simulink model "code_gen_man_bin"  (Simulink 7.5)
settings: Solver=FixedStepDiscrete  SolverMode=SingleTasking  StartTime=0.0  StopTime=10.0  FixedStep=0.01  RelTol=1e-3
InitFcn:
  | boat_constants
values from neighbouring files (symbols this model uses):
  figure8_waypoints = int32([ ... (first row only)    [boat_constants.m]
  InitialPoint = 0    [boat_constants.m]    (also in l2plus.m)
  IPStar = 0    [boat_constants.m]    (also in l2plus.m)
  ISA_g = 9.815    [boat_constants.m]
  MaxDwnPthStar = 1    [boat_constants.m]    (also in l2plus.m)
  OC2max = 49999    [boat_constants.m]    (also in simulation_constants.m)
  sampling_waypoints = int32([ ... (first row only)    [boat_constants.m]
  switchDistance = 4    [boat_constants.m]    (also in l2plus.m)
  T_step = 0.01    [boat_constants.m]    (also in common.m)
  tanIntercept = tan( 45*pi/180 )    [boat_constants.m]    (also in l2plus.m)
  test_waypoints = int32([ ... (first row only)    [boat_constants.m]
  TStar = single(4.5)    [boat_constants.m]    (also in l2plus.m = single(2))
  Turn2Track = 0    [boat_constants.m]    (also in l2plus.m)
  wheelbase = 3.27    [boat_constants.m]
undefined symbols (not defined in the file or in its folder): clearGpsData, clearSensorData, cpInitCommunications, DataEEInitAndClear, DataEEWrite, DiscIntNeverNeededParam, ecan1_buffered_transmit_matlab, ecan1_error_status_matlab, ecan1_init, GetAirData, getGpsData, getRevoData, getSensorData, GetThrottleData, GetWaterData, GetWindData, Init_onlyOnce, Init_Reset, initCalibrationRange, initGps, processNewCommData, processNewGpsData, processNewRevoData, setHilMode, u1, u2, uart1EnqueueStateData, uart2EnqueueActuatorData, y1
libraries: simulink x80, dsPICdrivers x50, uSimLib x4, simulink_need_slupdate x4
(part 2 of 6)

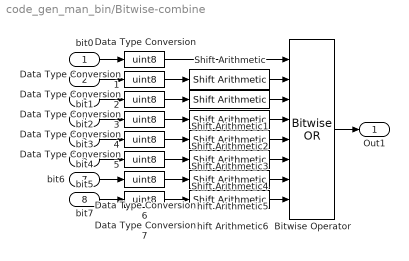
== system code_gen_man_bin/Bitwise-combine ==
  bit0 : Inport
  bit1 : Inport  Port=2
  bit2 : Inport  Port=3
  bit3 : Inport  Port=4
  bit4 : Inport  Port=5
  bit5 : Inport  Port=6
  bit6 : Inport  Port=7
  bit7 : Inport  Port=8
  Bitwise Operator : simulink/Logic and Bit Operations/Bitwise Operator  logicop=OR  UseBitMask=off  NumInputPorts=8  BitMask=bin2dec('11011001')  BitMaskRealWorld=Stored Integer
  Data Type Conversion{,1..7} (8 alike) : DataTypeConversion  OutDataTypeMode=uint8  OutDataType=fixdt(1, 16)  OutScaling=2^0  OutDataTypeStr=uint8
  Shift Arithmetic : simulink/Logic and Bit Operations/Shift Arithmetic  SystemSampleTime=-1  nBitShiftRight=-1  nBinPtShiftRight=0
  Shift Arithmetic1 : simulink/Logic and Bit Operations/Shift Arithmetic  SystemSampleTime=-1  nBitShiftRight=-2  nBinPtShiftRight=0
  Shift Arithmetic2 : simulink/Logic and Bit Operations/Shift Arithmetic  SystemSampleTime=-1  nBitShiftRight=-3  nBinPtShiftRight=0
  Shift Arithmetic3 : simulink/Logic and Bit Operations/Shift Arithmetic  SystemSampleTime=-1  nBitShiftRight=-4  nBinPtShiftRight=0
  Shift Arithmetic4 : simulink/Logic and Bit Operations/Shift Arithmetic  SystemSampleTime=-1  nBitShiftRight=-5  nBinPtShiftRight=0
  Shift Arithmetic5 : simulink/Logic and Bit Operations/Shift Arithmetic  SystemSampleTime=-1  nBitShiftRight=-6  nBinPtShiftRight=0
  Shift Arithmetic6 : simulink/Logic and Bit Operations/Shift Arithmetic  SystemSampleTime=-1  nBitShiftRight=-7  nBinPtShiftRight=0
  Out1 : Outport
  wires:
  Shift Arithmetic/1 -> Bitwise Operator/2
  Shift Arithmetic1/1 -> Bitwise Operator/3
  Shift Arithmetic2/1 -> Bitwise Operator/4
  Data Type Conversion/1 -> Bitwise Operator/1
  Data Type Conversion1/1 -> Shift Arithmetic/1
  Data Type Conversion2/1 -> Shift Arithmetic1/1
  Data Type Conversion3/1 -> Shift Arithmetic2/1
  Data Type Conversion4/1 -> Shift Arithmetic3/1
  Shift Arithmetic3/1 -> Bitwise Operator/5
  Data Type Conversion5/1 -> Shift Arithmetic4/1
  Data Type Conversion6/1 -> Shift Arithmetic5/1
  Shift Arithmetic4/1 -> Bitwise Operator/6
  Shift Arithmetic5/1 -> Bitwise Operator/7
  Data Type Conversion7/1 -> Shift Arithmetic6/1
  Shift Arithmetic6/1 -> Bitwise Operator/8
  bit0/1 -> Data Type Conversion/1
  bit1/1 -> Data Type Conversion1/1
  bit2/1 -> Data Type Conversion2/1
  bit3/1 -> Data Type Conversion3/1
  Bitwise Operator/1 -> Out1/1
  bit4/1 -> Data Type Conversion4/1
  bit5/1 -> Data Type Conversion5/1
  bit6/1 -> Data Type Conversion6/1
  bit7/1 -> Data Type Conversion7/1

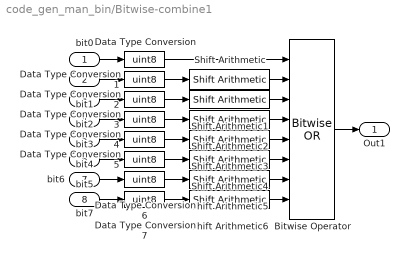
== system code_gen_man_bin/Bitwise-combine1 ==
  bit0 : Inport
  bit1 : Inport  Port=2
  bit2 : Inport  Port=3
  bit3 : Inport  Port=4
  bit4 : Inport  Port=5
  bit5 : Inport  Port=6
  bit6 : Inport  Port=7
  bit7 : Inport  Port=8
  Bitwise Operator : simulink/Logic and Bit Operations/Bitwise Operator  logicop=OR  UseBitMask=off  NumInputPorts=8  BitMask=bin2dec('11011001')  BitMaskRealWorld=Stored Integer
  Data Type Conversion{,1..7} (8 alike) : DataTypeConversion  OutDataTypeMode=uint8  OutDataType=fixdt(1, 16)  OutScaling=2^0  OutDataTypeStr=uint8
  Shift Arithmetic : simulink/Logic and Bit Operations/Shift Arithmetic  SystemSampleTime=-1  nBitShiftRight=-1  nBinPtShiftRight=0
  Shift Arithmetic1 : simulink/Logic and Bit Operations/Shift Arithmetic  SystemSampleTime=-1  nBitShiftRight=-2  nBinPtShiftRight=0
  Shift Arithmetic2 : simulink/Logic and Bit Operations/Shift Arithmetic  SystemSampleTime=-1  nBitShiftRight=-3  nBinPtShiftRight=0
  Shift Arithmetic3 : simulink/Logic and Bit Operations/Shift Arithmetic  SystemSampleTime=-1  nBitShiftRight=-4  nBinPtShiftRight=0
  Shift Arithmetic4 : simulink/Logic and Bit Operations/Shift Arithmetic  SystemSampleTime=-1  nBitShiftRight=-5  nBinPtShiftRight=0
  Shift Arithmetic5 : simulink/Logic and Bit Operations/Shift Arithmetic  SystemSampleTime=-1  nBitShiftRight=-6  nBinPtShiftRight=0
  Shift Arithmetic6 : simulink/Logic and Bit Operations/Shift Arithmetic  SystemSampleTime=-1  nBitShiftRight=-7  nBinPtShiftRight=0
  Out1 : Outport
  wires:
  Shift Arithmetic/1 -> Bitwise Operator/2
  Shift Arithmetic1/1 -> Bitwise Operator/3
  Shift Arithmetic2/1 -> Bitwise Operator/4
  Data Type Conversion/1 -> Bitwise Operator/1
  Data Type Conversion1/1 -> Shift Arithmetic/1
  Data Type Conversion2/1 -> Shift Arithmetic1/1
  Data Type Conversion3/1 -> Shift Arithmetic2/1
  Data Type Conversion4/1 -> Shift Arithmetic3/1
  Shift Arithmetic3/1 -> Bitwise Operator/5
  Data Type Conversion5/1 -> Shift Arithmetic4/1
  Data Type Conversion6/1 -> Shift Arithmetic5/1
  Shift Arithmetic4/1 -> Bitwise Operator/6
  Shift Arithmetic5/1 -> Bitwise Operator/7
  Data Type Conversion7/1 -> Shift Arithmetic6/1
  Shift Arithmetic6/1 -> Bitwise Operator/8
  bit0/1 -> Data Type Conversion/1
  bit1/1 -> Data Type Conversion1/1
  bit2/1 -> Data Type Conversion2/1
  bit3/1 -> Data Type Conversion3/1
  Bitwise Operator/1 -> Out1/1
  bit4/1 -> Data Type Conversion4/1
  bit5/1 -> Data Type Conversion5/1
  bit6/1 -> Data Type Conversion6/1
  bit7/1 -> Data Type Conversion7/1

== system code_gen_man_bin/Blink LED D10 a 1Hz ==
  Data Type Conversion : DataTypeConversion  OutDataTypeMode=boolean  OutDataType=sfix(16)  OutScaling=2^0  OutDataTypeStr=boolean  RndMeth=Simplest
  Repeating Sequence Stair : simulink/Sources/Repeating Sequence Stair  SystemSampleTime=-1  OutValues=[1 0]  tsamp=1  OutMin=[]  OutMax=[]  OutDataTypeStr=double  OutputDataTypeScalingMode=double  OutDataType=fixdt(0,8)  ConRadixGroup=Best Precision: Vector-wise  OutScaling=2^-12
  Running status (LED D10) : dsPICdrivers/Digital I//O/Digital Output Write  Tag=dsPIC_Digital_Output  Priority=5  PORT=A  Pin=[7]  Simultaneous=off  OrderingInOutPopup=None
  wires:
  Repeating Sequence Stair/1 -> Data Type Conversion/1
  Data Type Conversion/1 -> Running status (LED D10)/1

== system code_gen_man_bin/Configure ECAN 1 ==
  C Function Call [ecanFunctions.c] : dsPICdrivers/OTHERS/C Function Call  Tag=dsPIC_dsPIC_CFunctionCall  FctUpdate=Output Function  fctName='ecan1_init'  INPUT_SIZE=53  INPUT1=uint16  INPUT2=--  INPUT3=--  OUTPUT_SIZE=1  OUTPUT1=--  SampleTime=Inf  InputType=[ 4 ]  OutputType=[ ]  FctDeclaration=extern void ecan1_init(uint16_T* u1);  FctCall=ecan1_init(*%u1);  OrderingInOutPopup=None  FctStart=None  FctStart_Name=Init_onlyOnce  FctStart_Declaration=inline extern void Init_onlyOnce();  FctStart_Call=Init_onlyOnce();  FctInit=None  FctInit_Name=Init_Reset  FctInit_Declaration=inline extern void Init_Reset();  FctInit_Call=Init_Reset();  PinDigitalInput=[]  PinDigitalOutput=[]  AnalogueInput=[]
  Constant : Constant  Value=parameters  OutDataTypeMode=uint16  OutDataType=sfix(16)  OutScaling=2^0  OutDataTypeStr=uint16
  wires:
  Constant/1 -> C Function Call [ecanFunctions.c]/1

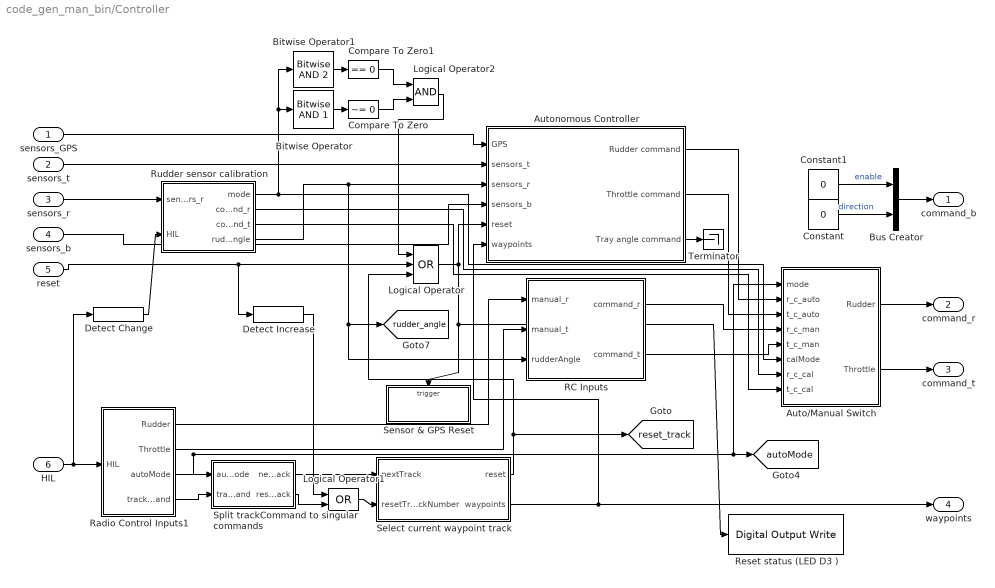
== system code_gen_man_bin/Controller ==
  sensors_GPS : Inport
  sensors_t : Inport  Port=2
  sensors_r : Inport  Port=3
  sensors_b : Inport  Port=4
  reset : Inport  Port=5
  HIL : Inport  Port=6
  Auto/Manual Switch : Subsystem
  Autonomous Controller : Subsystem
  Bitwise Operator : simulink/Logic and Bit Operations/Bitwise Operator  logicop=AND  UseBitMask=on  BitMask=1  BitMaskRealWorld=Stored Integer
  Bitwise Operator1 : simulink/Logic and Bit Operations/Bitwise Operator  logicop=AND  UseBitMask=on  BitMask=2  BitMaskRealWorld=Stored Integer
  Bus Creator : BusCreator  Inputs=2
  Compare To Zero : simulink/Logic and Bit Operations/Compare To Zero  SystemSampleTime=-1  relop=~=  LogicOutDataTypeMode=boolean
  Compare To Zero1 : simulink/Logic and Bit Operations/Compare To Zero  SystemSampleTime=-1  relop===  LogicOutDataTypeMode=boolean
  Constant : Constant  Value=0  OutDataTypeMode=boolean  OutDataType=fixdt(1, 16)  OutScaling=2^0  OutDataTypeStr=boolean
  Constant1 : Constant  Value=0  OutDataTypeMode=boolean  OutDataType=fixdt(1, 16)  OutScaling=2^0  OutDataTypeStr=boolean
  Detect Change : simulink/Logic and Bit Operations/Detect Change  SystemSampleTime=-1  vinit=0
  Detect Increase : simulink/Logic and Bit Operations/Detect Increase  SystemSampleTime=-1  vinit=0.0
  Logical Operator : Logic  Operator=OR  Inputs=3  AllPortsSameDT=off  OutDataTypeMode=boolean  LogicDataType=fixdt(0, 8)  OutDataTypeStr=boolean
  Logical Operator1 : Logic  Operator=OR  AllPortsSameDT=off  OutDataTypeMode=boolean  LogicDataType=fixdt(0, 8)  OutDataTypeStr=boolean
  Logical Operator2 : Logic  AllPortsSameDT=off  OutDataTypeMode=boolean  LogicDataType=fixdt(0, 8)  OutDataTypeStr=boolean
  RC Inputs : Subsystem
  Radio Control Inputs1 : Subsystem
  Reset status (LED D3 ) : dsPICdrivers/Digital I//O/Digital Output Write  Tag=dsPIC_Digital_Output  Priority=5  PORT=A  Pin=[0]  Simultaneous=off  OrderingInOutPopup=None
  Rudder sensor calibration : Subsystem
  Select current waypoint track : Stateflow chart  TreatAsAtomicUnit=on
  Sensor & GPS Reset : Subsystem
  Split trackCommand to singular commands : Subsystem
  Terminator : Terminator
  command_b : Outport
  command_r : Outport  Port=2
  command_t : Outport  Port=3
  waypoints : Outport  Port=4
  tag scope: autoMode=global, reset_track=global, rudder_angle=global
  wires:
  sensors_t/1 -> Autonomous Controller/2(sensors_t)
  sensors_GPS/1 -> Autonomous Controller/1(GPS)
  sensors_b/1 -> Autonomous Controller/4(sensors_b)
  Constant/1 -> Bus Creator/2  "direction"
  Bus Creator/1 -> command_b/1
  Constant1/1 -> Bus Creator/1  "enable"
  Autonomous Controller/3(Tray angle command) -> Terminator/1
  Radio Control Inputs1/3(autoMode) -> Split trackCommand to singular commands/1(autoMode), Auto/Manual Switch/1(mode), [autoMode]
  Radio Control Inputs1/1(Rudder) -> RC Inputs/1(manual_r)
  Radio Control Inputs1/2(Throttle) -> RC Inputs/2(manual_t)
  Select current waypoint track/1(reset) -> [reset_track], Logical Operator/3
  Logical Operator/1 -> Reset status (LED D3 )/1, Sensor & GPS Reset/Trigger, Autonomous Controller/5(reset)
  reset/1 -> Logical Operator/2, Detect Increase/1
  Split trackCommand to singular commands/1(nextTrack) -> Select current waypoint track/1(nextTrack)
  Radio Control Inputs1/4(trackCommand) -> Split trackCommand to singular commands/2(trackCommand)
  Autonomous Controller/1(Rudder command) -> Auto/Manual Switch/2(r_c_auto)
  Autonomous Controller/2(Throttle command) -> Auto/Manual Switch/3(t_c_auto)
  RC Inputs/1(command_r) -> Auto/Manual Switch/4(r_c_man)
  RC Inputs/2(command_t) -> Auto/Manual Switch/5(t_c_man)
  Auto/Manual Switch/1(Rudder) -> command_r/1
  Auto/Manual Switch/2(Throttle) -> command_t/1
  Select current waypoint track/2(waypoints) -> waypoints/1, Autonomous Controller/6(waypoints)
  Split trackCommand to singular commands/2(resetTrack) -> Logical Operator1/2
  Logical Operator1/1 -> Select current waypoint track/2(resetTrackNumber)
  Rudder sensor calibration/4(rudderAngle) -> RC Inputs/3(rudderAngle), [rudder_angle], Autonomous Controller/3(sensors_r)
  HIL/1 -> Detect Change/1, Radio Control Inputs1/1(HIL)
  Detect Increase/1 -> Logical Operator1/1
  Rudder sensor calibration/1(mode) -> Auto/Manual Switch/6(calMode), Bitwise Operator/1, Bitwise Operator1/1
  Rudder sensor calibration/2(command_r) -> Auto/Manual Switch/7(r_c_cal)
  Rudder sensor calibration/3(command_t) -> Auto/Manual Switch/8(t_c_cal)
  Bitwise Operator/1 -> Compare To Zero/1
  sensors_r/1 -> Rudder sensor calibration/1(sensors_r)
  Detect Change/1 -> Rudder sensor calibration/2(HIL)
  Compare To Zero/1 -> Logical Operator2/2
  Compare To Zero1/1 -> Logical Operator2/1
  Logical Operator2/1 -> Logical Operator/1
  Bitwise Operator1/1 -> Compare To Zero1/1

== system code_gen_man_bin/ECAN1 Error Status ==
  C Function Call [ecanFunctions.c] : dsPICdrivers/OTHERS/C Function Call  Tag=dsPIC_dsPIC_CFunctionCall  FctUpdate=Output Function  fctName='ecan1_error_status_matlab'  INPUT_SIZE=1  INPUT1=--  INPUT2=--  INPUT3=--  OUTPUT_SIZE=2  OUTPUT1=uint8  SampleTime=ecan1_error_sample_time  InputType=[ ]  OutputType=[ 2 ]  FctDeclaration=extern void ecan1_error_status_matlab(uint8_T* y1);  FctCall=ecan1_error_status_matlab(*%y1);  OrderingInOutPopup=None  FctStart=None  FctStart_Name=Init_onlyOnce  FctStart_Declaration=inline extern void Init_onlyOnce();  FctStart_Call=Init_onlyOnce();  FctInit=None  FctInit_Name=Init_Reset  FctInit_Declaration=inline extern void Init_Reset();  FctInit_Call=Init_Reset();  PinDigitalInput=[]  PinDigitalOutput=[]  AnalogueInput=[]
  Demux : Demux  Outputs=2
  tx_err : Outport  OutDataType=sfix(16)  OutScaling=2^0
  rx_err : Outport  Port=2  OutDataType=sfix(16)  OutScaling=2^0
  wires:
  Demux/2 -> rx_err/1
  Demux/1 -> tx_err/1
  C Function Call [ecanFunctions.c]/1 -> Demux/1

== system code_gen_man_bin/Load1 ==
  Calculus Time Step : dsPICdrivers/OTHERS/Calculus Time Step  Tag=dsPIC_CalculusTimeStep  SampleTime=0.01  PR1chk=on
  Compare To Zero : simulink/Logic and Bit Operations/Compare To Zero  SystemSampleTime=-1  relop=~=  LogicOutDataTypeMode=uint8
  Constant : Constant  OutDataType=fixdt(1, 16)  OutScaling=2^0
  Data Type Conversion5 : DataTypeConversion  OutDataTypeMode=uint8  OutDataTypeStr=uint8
  Data Type Conversion6 : DataTypeConversion  OutDataTypeMode=single  OutDataType=fixdt(1, 16)  OutScaling=2^0  OutDataTypeStr=single
  Data Type Conversion7 : DataTypeConversion  OutDataTypeMode=single  OutDataType=fixdt(1, 16)  OutScaling=2^0  OutDataTypeStr=single
  Gain : Gain  Gain=100
  Product : Product  Inputs=*/  RndMeth=Zero
  Switch : Switch  Criteria=u2 ~= 0  OutDataType=fixdt(1, 16)  OutScaling=2^0
  load : Outport
  wires:
  Calculus Time Step/1 -> Data Type Conversion6/1
  Calculus Time Step/2 -> Data Type Conversion7/1
  Product/1 -> Gain/1
  Gain/1 -> Data Type Conversion5/1
  Data Type Conversion6/1 -> Product/1
  Data Type Conversion5/1 -> load/1
  Data Type Conversion7/1 -> Switch/1, Compare To Zero/1
  Switch/1 -> Product/2
  Compare To Zero/1 -> Switch/2
  Constant/1 -> Switch/3

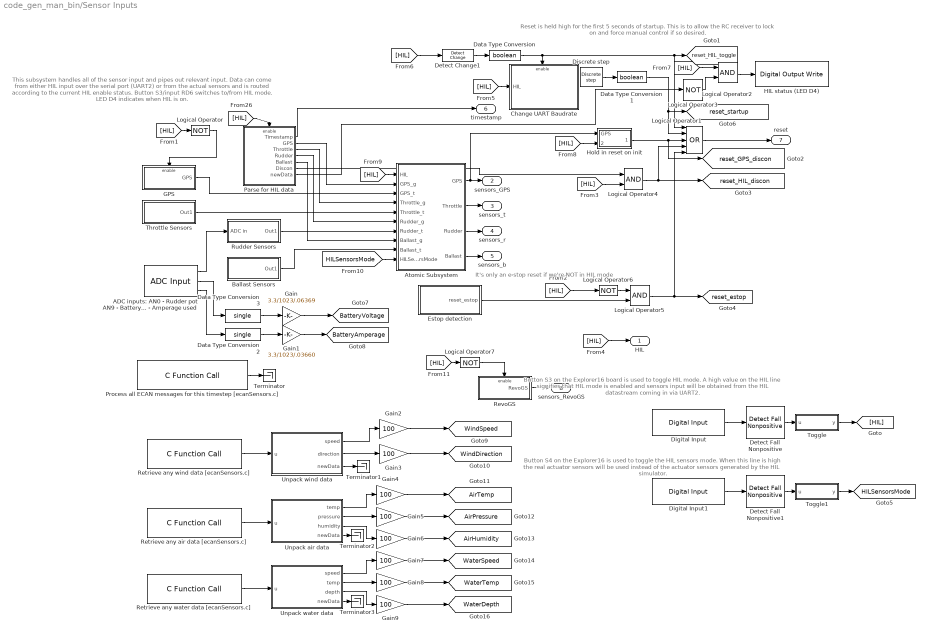
== system code_gen_man_bin/Sensor Inputs ==
  note: This subsystem handles all of the sensor input and pipes out relevant input. Data can come
      | from either HIL input over the serial port (UART2) or from the actual sensors and is routed
      | according to the current HIL enable status. Button S3/input RD6 switches to/from HIL mode.
      | LED D4 indicates when HIL is on.
  note: Reset is held high for the first 5 seconds of startup. This is to allow
      | the RC receiver to lock on and force manual control if so desired.
  note: It's only an e-stop reset if we're NOT in HIL mode
  note: Button S3 on the Explorer16 board is used to toggle HIL mode. A high value
      | on the HIL line signifies that HIL mode is enabled and sensors input will be
      | obtained from the HIL datastream coming in via UART2.
  note: Button S4 on the Explorer16 is used to toggle the HIL sensors mode.
      | When this line is high the real actuator sensors will be used
      | instead of the actuator sensors generated by the HIL simulator.
  ADC inputs: AN0 - Rudder pot AN9 - Battery voltage AN11 - Amperage used : dsPICdrivers/Peripheral I//O/ADC Input  Tag=dsPIC_ADC  Priority=5  ADC_TYPE=10 bits  ADC_MODE=Continuous sampling & get last channel value  NbrSampleStep=1  VoltRefpopup="AVdd  -  AVss"  OutFormatBitspopup=0000 00dd dddd dddd : Integer  InterruptPriority=6  ANCHANNELS=[0 9 11]  MaxName=ANmax = 1023  Rin=0  ADCS=12  SAMC=1  Temperature=25  DMAChannel=7  SampleTime=.01  Status="OK  |  Tsmp=1.625e-007 |  T/Channel=2.113e-006 |  Tall=6.337e-006"  SSRC=auto convert
  Atomic Subsystem : Subsystem
  Ballast Sensors : Subsystem
  Change UART Baudrate : Subsystem
  Data Type Conversion : DataTypeConversion  OutDataTypeMode=boolean  OutDataType=fixdt(1, 16)  OutScaling=2^0  OutDataTypeStr=boolean
  Data Type Conversion1 : DataTypeConversion  OutDataTypeMode=boolean  OutDataType=fixdt(1, 16)  OutScaling=2^0  OutDataTypeStr=boolean
  Data Type Conversion2 : DataTypeConversion  OutDataTypeMode=single  OutDataType=fixdt(1, 16)  OutScaling=2^0  OutDataTypeStr=single
  Data Type Conversion3 : DataTypeConversion  OutDataTypeMode=single  OutDataType=fixdt(1, 16)  OutScaling=2^0  OutDataTypeStr=single
  Detect Change1 : simulink/Logic and Bit Operations/Detect Change  SystemSampleTime=-1  vinit=0
  Detect Fall Nonpositive : simulink/Logic and Bit Operations/Detect Fall Nonpositive  SystemSampleTime=-1  vinit=1
  Detect Fall Nonpositive1 : simulink/Logic and Bit Operations/Detect Fall Nonpositive  SystemSampleTime=-1  vinit=1
  Digital Input : dsPICdrivers/Digital I//O/Digital Input  Tag=dsPIC_Digital_Input  PORT=D  Pin=[6]  SampleTime=T_step  OrderingInOutPopup=None
  Digital Input1 : dsPICdrivers/Digital I//O/Digital Input  Tag=dsPIC_Digital_Input  PORT=D  Pin=[13]  SampleTime=T_step  OrderingInOutPopup=None
  Discrete step : uSimLib/Sources/Discrete step  SystemSampleTime=-1  start_value=1  end_value=0  transition_time=500
  Estop detection : Subsystem
  GPS : Subsystem
  Gain : Gain  Gain=3.3/1023/.06369  ParameterDataType=fixdt(1, 16)  ParameterScaling=2^0  OutDataType=fixdt(1, 16)  OutScaling=2^0
  Gain1 : Gain  Gain=3.3/1023/.03660  ParameterDataType=fixdt(1, 16)  ParameterScaling=2^0  OutDataType=fixdt(1, 16)  OutScaling=2^0
  Gain{2..3,5..7,9} (6 alike) : Gain  Gain=100  ParameterDataType=fixdt(1, 16)  ParameterScaling=2^0  OutDataTypeMode=uint16  OutDataType=fixdt(1, 16)  OutScaling=2^0  OutDataTypeStr=uint16
  Gain4 : Gain  Gain=100  ParameterDataType=fixdt(1, 16)  ParameterScaling=2^0  OutDataTypeMode=int16  OutDataType=fixdt(1, 16)  OutScaling=2^0  OutDataTypeStr=int16
  Gain8 : Gain  Gain=100  ParameterDataType=fixdt(1, 16)  ParameterScaling=2^0  OutDataTypeMode=int16  OutDataType=fixdt(1, 16)  OutScaling=2^0  OutDataTypeStr=int16
  HIL status (LED D4) : dsPICdrivers/Digital I//O/Digital Output Write  Tag=dsPIC_Digital_Output  Priority=5  PORT=A  Pin=[1]  Simultaneous=off  OrderingInOutPopup=None
  Hold in reset on init : Subsystem
  Logical Operator : Logic  Operator=NOT  AllPortsSameDT=off  OutDataTypeMode=boolean  LogicDataType=fixdt(0, 8)  OutDataTypeStr=boolean
  Logical Operator1 : Logic  Operator=OR  Inputs=5  AllPortsSameDT=off  OutDataTypeMode=boolean  LogicDataType=fixdt(0, 8)  OutDataTypeStr=boolean
  Logical Operator2 : Logic  AllPortsSameDT=off  OutDataTypeMode=boolean  LogicDataType=fixdt(0, 8)  OutDataTypeStr=boolean
  Logical Operator3 : Logic  Operator=NOT  Inputs=1  AllPortsSameDT=off  OutDataTypeMode=boolean  LogicDataType=fixdt(0, 8)  OutDataTypeStr=boolean
  Logical Operator4 : Logic  AllPortsSameDT=off  OutDataTypeMode=boolean  LogicDataType=fixdt(0, 8)  OutDataTypeStr=boolean
  Logical Operator5 : Logic  AllPortsSameDT=off  OutDataTypeMode=boolean  LogicDataType=fixdt(0, 8)  OutDataTypeStr=boolean
  Logical Operator6 : Logic  Operator=NOT  AllPortsSameDT=off  OutDataTypeMode=boolean  LogicDataType=fixdt(0, 8)  OutDataTypeStr=boolean
  Logical Operator7 : Logic  Operator=NOT  AllPortsSameDT=off  OutDataTypeMode=boolean  LogicDataType=fixdt(0, 8)  OutDataTypeStr=boolean
  Parse for HIL data : Subsystem
  Process all ECAN messages for this timestep [ecanSensors.c] : dsPICdrivers/OTHERS/C Function Call  Tag=dsPIC_dsPIC_CFunctionCall  FctUpdate=Output Function  fctName=ProcessAllEcanMessages  INPUT_SIZE=1  INPUT1=--  INPUT2=--  INPUT3=--  OUTPUT_SIZE=1  OUTPUT1=uint8  SampleTime=.01  InputType=[ ]  OutputType=[ 2 ]  FctDeclaration=extern uint8_T ProcessAllEcanMessages();  FctCall=%y1 = ProcessAllEcanMessages();  OrderingInOutPopup=None  FctStart=None  FctStart_Name=Init_onlyOnce  FctStart_Declaration=inline extern void Init_onlyOnce();  FctStart_Call=Init_onlyOnce();  FctInit=None  FctInit_Name=Init_Reset  FctInit_Declaration=inline extern void Init_Reset();  FctInit_Call=Init_Reset();  PinDigitalInput=[]  PinDigitalOutput=[]  AnalogueInput=[]
  Retrieve any air data [ecanSensors.c] : dsPICdrivers/OTHERS/C Function Call  Tag=dsPIC_dsPIC_CFunctionCall  FctUpdate=Output Function  fctName=GetAirData  INPUT_SIZE=1  INPUT1=--  INPUT2=--  INPUT3=--  OUTPUT_SIZE=13  OUTPUT1=uint8  SampleTime=.01  InputType=[ ]  OutputType=[ 2 ]  FctDeclaration=extern void GetAirData(uint8_T* y1);  FctCall=GetAirData(*%y1);  OrderingInOutPopup=None  FctStart=None  FctStart_Name=Init_onlyOnce  FctStart_Declaration=inline extern void Init_onlyOnce();  FctStart_Call=Init_onlyOnce();  FctInit=None  FctInit_Name=Init_Reset  FctInit_Declaration=inline extern void Init_Reset();  FctInit_Call=Init_Reset();  PinDigitalInput=[]  PinDigitalOutput=[]  AnalogueInput=[]
  Retrieve any water data [ecanSensors.c] : dsPICdrivers/OTHERS/C Function Call  Tag=dsPIC_dsPIC_CFunctionCall  FctUpdate=Output Function  fctName=GetWaterData  INPUT_SIZE=1  INPUT1=--  INPUT2=--  INPUT3=--  OUTPUT_SIZE=13  OUTPUT1=uint8  SampleTime=.01  InputType=[ ]  OutputType=[ 2 ]  FctDeclaration=extern void GetWaterData(uint8_T* y1);  FctCall=GetWaterData(*%y1);  OrderingInOutPopup=None  FctStart=None  FctStart_Name=Init_onlyOnce  FctStart_Declaration=inline extern void Init_onlyOnce();  FctStart_Call=Init_onlyOnce();  FctInit=None  FctInit_Name=Init_Reset  FctInit_Declaration=inline extern void Init_Reset();  FctInit_Call=Init_Reset();  PinDigitalInput=[]  PinDigitalOutput=[]  AnalogueInput=[]
  Retrieve any wind data [ecanSensors.c] : dsPICdrivers/OTHERS/C Function Call  Tag=dsPIC_dsPIC_CFunctionCall  FctUpdate=Output Function  fctName=GetWindData  INPUT_SIZE=1  INPUT1=--  INPUT2=--  INPUT3=--  OUTPUT_SIZE=9  OUTPUT1=uint8  SampleTime=.01  InputType=[ ]  OutputType=[ 2 ]  FctDeclaration=extern void GetWindData(uint8_T* y1);  FctCall=GetWindData(*%y1);  OrderingInOutPopup=None  FctStart=None  FctStart_Name=Init_onlyOnce  FctStart_Declaration=inline extern void Init_onlyOnce();  FctStart_Call=Init_onlyOnce();  FctInit=None  FctInit_Name=Init_Reset  FctInit_Declaration=inline extern void Init_Reset();  FctInit_Call=Init_Reset();  PinDigitalInput=[]  PinDigitalOutput=[]  AnalogueInput=[]
  RevoGS : Subsystem
  Rudder Sensors : Subsystem
  Terminator{,1..3} (4 alike) : Terminator
  Throttle Sensors : Subsystem
  Toggle : Stateflow chart  TreatAsAtomicUnit=on
  Toggle1 : Stateflow chart  TreatAsAtomicUnit=on
  Unpack air data : Stateflow chart  TreatAsAtomicUnit=on
  Unpack water data : Stateflow chart  TreatAsAtomicUnit=on
  Unpack wind data : Stateflow chart  TreatAsAtomicUnit=on
  HIL : Outport
  sensors_GPS : Outport  Port=2
  sensors_t : Outport  Port=3
  sensors_r : Outport  Port=4
  sensors_b : Outport  Port=5
  timestamp : Outport  Port=6
  reset : Outport  Port=7
  sensors_RevoGS : Outport  Port=8
  tag scope: AirHumidity=global, AirPressure=global, AirTemp=global, BatteryAmperage=global, BatteryVoltage=global, HILSensorsMode=global, WaterDepth=global, WaterSpeed=global, WaterTemp=global, WindDirection=global, WindSpeed=global, reset_GPS_discon=global, reset_HIL_discon=global, reset_HIL_toggle=global, reset_estop=global, reset_startup=global
  wires:
  Rudder Sensors/1(Out1) -> Atomic Subsystem/7(Rudder_t)
  GPS/1(GPS) -> Atomic Subsystem/3(GPS_t)
  Throttle Sensors/1(Out1) -> Atomic Subsystem/5(Throttle_t)
  Ballast Sensors/1(Out1) -> Atomic Subsystem/9(Ballast_t)
  Parse for HIL data/2(GPS) -> Atomic Subsystem/2(GPS_g)
  Parse for HIL data/3(Throttle) -> Atomic Subsystem/4(Throttle_g)
  Parse for HIL data/4(Rudder) -> Atomic Subsystem/6(Rudder_g)
  Parse for HIL data/5(Ballast) -> Atomic Subsystem/8(Ballast_g)
  Atomic Subsystem/2(Throttle) -> sensors_t/1
  Atomic Subsystem/3(Rudder) -> sensors_r/1
  Atomic Subsystem/4(Ballast) -> sensors_b/1
  Atomic Subsystem/1(GPS) -> sensors_GPS/1, Hold in reset on init/1(GPS)
  Parse for HIL data/1(Timestamp) -> timestamp/1
  Digital Input/1 -> Detect Fall Nonpositive/1
  Detect Fall Nonpositive/1 -> Toggle/1(u)
  Detect Change1/1 -> Data Type Conversion/1
  Logical Operator/1 -> GPS/Enable
  Logical Operator1/1 -> reset/1
  Discrete step/1 -> Data Type Conversion1/1
  Hold in reset on init/1(Out1) -> Logical Operator1/3, [reset_GPS_discon]
  Parse for HIL data/6(Discon) -> Logical Operator4/1
  Data Type Conversion/1 -> Change UART Baudrate/Enable, Logical Operator1/1, [reset_HIL_toggle]
  Data Type Conversion1/1 -> Logical Operator1/2, [reset_startup]
  Logical Operator2/1 -> HIL status (LED D4)/1
  Logical Operator3/1 -> Logical Operator2/2
  Parse for HIL data/7(newData) -> Logical Operator3/1
  Logical Operator4/1 -> Logical Operator1/4, [reset_HIL_discon]
  Estop detection/1(reset_estop) -> Logical Operator5/2
  Logical Operator5/1 -> [reset_estop], Logical Operator1/5
  Logical Operator6/1 -> Logical Operator5/1
  Toggle/1(y) -> [HIL]
  [HIL] -> Parse for HIL data/Enable
  [HIL] -> Logical Operator/1
  [HIL] -> Logical Operator6/1
  [HIL] -> Logical Operator4/2
  [HIL] -> HIL/1
  [HIL] -> Change UART Baudrate/1(HIL)
  [HIL] -> Detect Change1/1
  [HIL] -> Logical Operator2/1
  [HIL] -> Hold in reset on init/2(HIL Button)
  [HIL] -> Atomic Subsystem/1(HIL)
  ADC inputs: AN0 - Rudder pot AN9 - Battery voltage AN11 - Amperage used/1 -> Rudder Sensors/1(ADC in)
  Digital Input1/1 -> Detect Fall Nonpositive1/1
  Detect Fall Nonpositive1/1 -> Toggle1/1(u)
  Toggle1/1(y) -> [HILSensorsMode]
  [HILSensorsMode] -> Atomic Subsystem/10(HILSensorsMode)
  Gain1/1 -> [BatteryAmperage]
  Gain/1 -> [BatteryVoltage]
  Data Type Conversion3/1 -> Gain/1
  Data Type Conversion2/1 -> Gain1/1
  ADC inputs: AN0 - Rudder pot AN9 - Battery voltage AN11 - Amperage used/2 -> Data Type Conversion3/1
  ADC inputs: AN0 - Rudder pot AN9 - Battery voltage AN11 - Amperage used/3 -> Data Type Conversion2/1
  [HIL] -> Logical Operator7/1
  Logical Operator7/1 -> RevoGS/Enable
  RevoGS/1(RevoGS) -> sensors_RevoGS/1
  Process all ECAN messages for this timestep [ecanSensors.c]/1 -> Terminator/1
  Retrieve any wind data [ecanSensors.c]/1 -> Unpack wind data/1(u)
  Unpack wind data/1(speed) -> Gain2/1
  Unpack wind data/2(direction) -> Gain3/1
  Unpack wind data/3(newData) -> Terminator1/1
  Retrieve any air data [ecanSensors.c]/1 -> Unpack air data/1(u)
  Retrieve any water data [ecanSensors.c]/1 -> Unpack water data/1(u)
  Unpack air data/1(temp) -> Gain4/1
  Unpack air data/2(pressure) -> Gain5/1
  Unpack air data/3(humidity) -> Gain6/1
  Unpack air data/4(newData) -> Terminator2/1
  Unpack water data/1(speed) -> Gain7/1
  Unpack water data/2(temp) -> Gain8/1
  Unpack water data/3(depth) -> Gain9/1
  Unpack water data/4(newData) -> Terminator3/1
  Gain2/1 -> [WindSpeed]
  Gain3/1 -> [WindDirection]
  Gain4/1 -> [AirTemp]
  Gain5/1 -> [AirPressure]
  Gain6/1 -> [AirHumidity]
  Gain7/1 -> [WaterSpeed]
  Gain8/1 -> [WaterTemp]
  Gain9/1 -> [WaterDepth]

== system code_gen_man_bin/Transmit actuator data ==
  rudder : Inport  OutDataType=fixdt(1, 16)  OutScaling=2^0
  throttle : Inport  Port=2  OutDataType=fixdt(1, 16)  OutScaling=2^0
  ballast : Inport  Port=3  OutDataType=fixdt(1, 16)  OutScaling=2^0
  seconds : Inport  Port=4  OutDataType=fixdt(1, 16)  OutScaling=2^0
  HIL enable : Inport  Port=5  OutDataType=fixdt(1, 16)  OutScaling=2^0
  rudderAngle : Inport  Port=6  OutDataType=fixdt(1, 16)  OutScaling=2^0
  sensorOverride : Inport  Port=7  OutDataType=fixdt(1, 16)  OutScaling=2^0
  Package and Transmit Sensor Struct : Subsystem
  wires:
  rudder/1 -> Package and Transmit Sensor Struct/1(command_r)
  throttle/1 -> Package and Transmit Sensor Struct/3(command_t)
  ballast/1 -> Package and Transmit Sensor Struct/2(command_b)
  seconds/1 -> Package and Transmit Sensor Struct/4(timstamp)
  HIL enable/1 -> Package and Transmit Sensor Struct/Enable
  rudderAngle/1 -> Package and Transmit Sensor Struct/5(rudderAngle)
  sensorOverride/1 -> Package and Transmit Sensor Struct/6(sensorOverride)

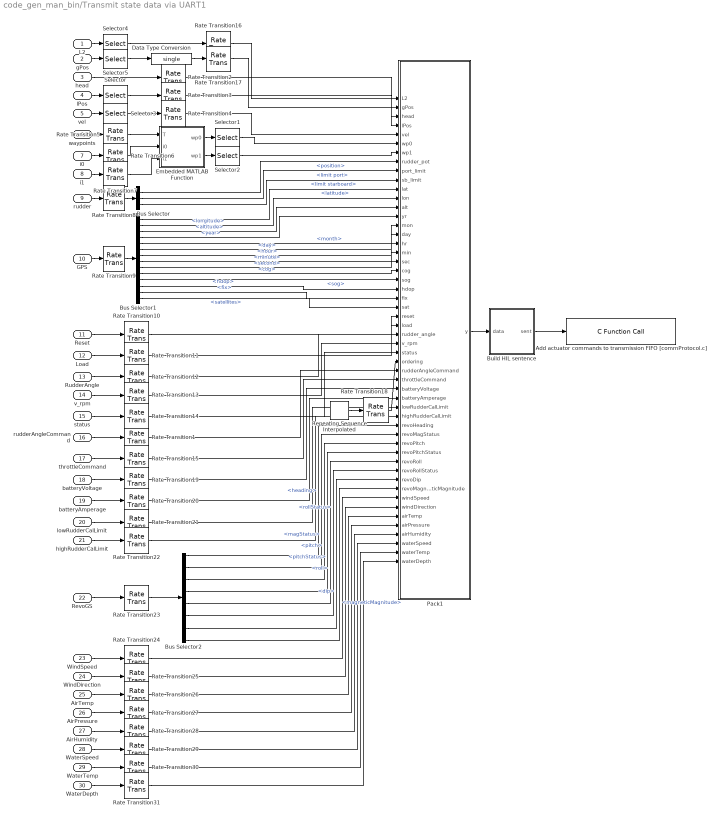
== system code_gen_man_bin/Transmit state data via UART1 ==
  L2 : Inport
  gPos : Inport  Port=2
  head : Inport  Port=3
  lPos : Inport  Port=4
  vel : Inport  Port=5
  waypoints : Inport  Port=6
  i0 : Inport  Port=7
  i1 : Inport  Port=8
  rudder : Inport  Port=9
  GPS : Inport  Port=10
  Reset : Inport  Port=11
  Load : Inport  Port=12
  RudderAngle : Inport  Port=13
  v_rpm : Inport  Port=14
  status : Inport  Port=15
  rudderAngleCommand : Inport  Port=16
  throttleCommand : Inport  Port=17
  batteryVoltage : Inport  Port=18
  batteryAmperage : Inport  Port=19
  lowRudderCalLimit : Inport  Port=20
  highRudderCalLimit : Inport  Port=21
  RevoGS : Inport  Port=22
  WindSpeed : Inport  Port=23
  WindDirection : Inport  Port=24
  AirTemp : Inport  Port=25
  AirPressure : Inport  Port=26
  AirHumidity : Inport  Port=27
  WaterSpeed : Inport  Port=28
  WaterTemp : Inport  Port=29
  WaterDepth : Inport  Port=30
  Add actuator commands to transmission FIFO [commProtocol.c] : dsPICdrivers/OTHERS/C Function Call  Tag=dsPIC_dsPIC_CFunctionCall  FctUpdate=Output Function  fctName='uart1EnqueueStateData'  INPUT_SIZE=160  INPUT1=uint8  INPUT2=--  INPUT3=--  OUTPUT_SIZE=1  OUTPUT1=--  SampleTime=-1  InputType=[ 2 ]  OutputType=[ ]  FctDeclaration=extern void uart1EnqueueStateData(uint8_T* u1);  FctCall=uart1EnqueueStateData(*%u1);  OrderingInOutPopup=None  FctStart=None  FctStart_Name=Init_onlyOnce  FctStart_Declaration=inline extern void Init_onlyOnce();  FctStart_Call=Init_onlyOnce();  FctInit=None  FctInit_Name=Init_Reset  FctInit_Declaration=inline extern void Init_Reset();  FctInit_Call=Init_Reset();  PinDigitalInput=[]  PinDigitalOutput=[]  AnalogueInput=[]
  Build HIL sentence : Subsystem
  Bus Selector : BusSelector  OutputSignals=position,limit port,limit starboard
  Bus Selector1 : BusSelector  OutputSignals=latitude,longitude,altitude,year,month,day,hour,minute,second,cog,sog,hdop,fix,satellites
  Bus Selector2 : BusSelector  OutputSignals=heading,magStatus,pitch,pitchStatus,roll,rollStatus,dip,magneticMagnitude
  Data Type Conversion : DataTypeConversion  OutDataTypeMode=single  OutDataType=fixdt(1, 16)  OutScaling=2^0  OutDataTypeStr=single
  Embedded MATLAB Function : Stateflow chart  TreatAsAtomicUnit=on
  Pack1 : Stateflow chart  TreatAsAtomicUnit=on
  Rate Transition{1..31} (31 alike) : RateTransition  OutPortSampleTime=telemetryDataRate
  Repeating Sequence Interpolated : simulink/Sources/Repeating Sequence Interpolated  SystemSampleTime=-1  OutValues=[0 255]  TimeValues=[0 2.55]  LookUpMeth=Interpolation-Use End Values  tsamp=T_step  OutMin=[]  OutMax=[]  OutDataTypeStr=uint8  OutputDataTypeScalingMode=uint8  OutDataType=fixdt(0,8)  OutScaling=2^-10
  Selector{,1..5} (6 alike) : Selector  InputPortWidth=3  IndexOptions=Index vector (dialog)  Indices=[1 2]  OutputSizes=1
  wires:
  Pack1/1(y) -> Build HIL sentence/1(data)
  Build HIL sentence/1(sent) -> Add actuator commands to transmission FIFO [commProtocol.c]/1
  gPos/1 -> Selector5/1
  i0/1 -> Rate Transition6/1
  waypoints/1 -> Rate Transition5/1
  i1/1 -> Rate Transition7/1
  Embedded MATLAB Function/1(wp0) -> Selector1/1
  Embedded MATLAB Function/2(wp1) -> Selector2/1
  rudder/1 -> Rate Transition8/1
  GPS/1 -> Rate Transition9/1
  L2/1 -> Selector4/1
  Data Type Conversion/1 -> Rate Transition17/1
  head/1 -> Rate Transition2/1
  lPos/1 -> Selector/1
  vel/1 -> Selector3/1
  Selector1/1 -> Pack1/6(wp0)
  Selector2/1 -> Pack1/7(wp1)
  Bus Selector/1 -> Pack1/8(rudder_pot)  "<position>"
  Bus Selector/2 -> Pack1/9(port_limit)  "<limit port>"
  Bus Selector/3 -> Pack1/10(sb_limit)  "<limit starboard>"
  Bus Selector1/1 -> Pack1/11(lat)  "<latitude>"
  Bus Selector1/2 -> Pack1/12(lon)  "<longitude>"
  Bus Selector1/3 -> Pack1/13(alt)  "<altitude>"
  Bus Selector1/4 -> Pack1/14(yr)  "<year>"
  Bus Selector1/5 -> Pack1/15(mon)  "<month>"
  Bus Selector1/6 -> Pack1/16(day)  "<day>"
  Bus Selector1/7 -> Pack1/17(hr)  "<hour>"
  Bus Selector1/8 -> Pack1/18(min)  "<minute>"
  Bus Selector1/9 -> Pack1/19(sec)  "<second>"
  Bus Selector1/10 -> Pack1/20(cog)  "<cog>"
  Bus Selector1/11 -> Pack1/21(sog)  "<sog>"
  Bus Selector1/12 -> Pack1/22(hdop)  "<hdop>"
  Bus Selector1/13 -> Pack1/23(fix)  "<fix>"
  Bus Selector1/14 -> Pack1/24(sat)  "<satellites>"
  Reset/1 -> Rate Transition10/1
  Load/1 -> Rate Transition11/1
  RudderAngle/1 -> Rate Transition12/1
  v_rpm/1 -> Rate Transition13/1
  status/1 -> Rate Transition14/1
  Repeating Sequence Interpolated/1 -> Rate Transition18/1
  Rate Transition14/1 -> Pack1/29(status)
  Rate Transition13/1 -> Pack1/28(v_rpm)
  Rate Transition12/1 -> Pack1/27(rudder_angle)
  Rate Transition11/1 -> Pack1/26(load)
  Rate Transition10/1 -> Pack1/25(reset)
  Rate Transition9/1 -> Bus Selector1/1
  Rate Transition8/1 -> Bus Selector/1
  Rate Transition7/1 -> Embedded MATLAB Function/3(i1)
  Rate Transition5/1 -> Embedded MATLAB Function/1(T)
  Rate Transition6/1 -> Embedded MATLAB Function/2(i0)
  Rate Transition4/1 -> Pack1/5(vel)
  Rate Transition3/1 -> Pack1/4(lPos)
  Rate Transition2/1 -> Pack1/3(head)
  Selector5/1 -> Data Type Conversion/1
  Selector4/1 -> Rate Transition16/1
  Selector/1 -> Rate Transition3/1
  Selector3/1 -> Rate Transition4/1
  rudderAngleCommand/1 -> Rate Transition1/1
  Rate Transition1/1 -> Pack1/31(rudderAngleCommand)
  throttleCommand/1 -> Rate Transition15/1
  Rate Transition15/1 -> Pack1/32(throttleCommand)
  Rate Transition16/1 -> Pack1/1(L2)
  Rate Transition17/1 -> Pack1/2(gPos)
  Rate Transition18/1 -> Pack1/30(ordering)
  batteryVoltage/1 -> Rate Transition19/1
  batteryAmperage/1 -> Rate Transition20/1
  Rate Transition19/1 -> Pack1/33(batteryVoltage)
  Rate Transition20/1 -> Pack1/34(batteryAmperage)
  lowRudderCalLimit/1 -> Rate Transition21/1
  highRudderCalLimit/1 -> Rate Transition22/1
  Rate Transition21/1 -> Pack1/35(lowRudderCalLimit)
  Rate Transition22/1 -> Pack1/36(highRudderCalLimit)
  RevoGS/1 -> Rate Transition23/1
  Rate Transition23/1 -> Bus Selector2/1
  Bus Selector2/1 -> Pack1/37(revoHeading)  "<heading>"
  Bus Selector2/2 -> Pack1/38(revoMagStatus)  "<magStatus>"
  Bus Selector2/3 -> Pack1/39(revoPitch)  "<pitch>"
  Bus Selector2/4 -> Pack1/40(revoPitchStatus)  "<pitchStatus>"
  Bus Selector2/5 -> Pack1/41(revoRoll)  "<roll>"
  Bus Selector2/6 -> Pack1/42(revoRollStatus)  "<rollStatus>"
  Bus Selector2/7 -> Pack1/43(revoDip)  "<dip>"
  Bus Selector2/8 -> Pack1/44(revoMagneticMagnitude)  "<magneticMagnitude>"
  WindSpeed/1 -> Rate Transition24/1
  WaterDepth/1 -> Rate Transition31/1
  WaterTemp/1 -> Rate Transition30/1
  WaterSpeed/1 -> Rate Transition29/1
  AirHumidity/1 -> Rate Transition28/1
  AirPressure/1 -> Rate Transition27/1
  AirTemp/1 -> Rate Transition26/1
  WindDirection/1 -> Rate Transition25/1
  Rate Transition24/1 -> Pack1/45(windSpeed)
  Rate Transition25/1 -> Pack1/46(windDirection)
  Rate Transition26/1 -> Pack1/47(airTemp)
  Rate Transition27/1 -> Pack1/48(airPressure)
  Rate Transition28/1 -> Pack1/49(airHumidity)
  Rate Transition29/1 -> Pack1/50(waterSpeed)
  Rate Transition30/1 -> Pack1/51(waterTemp)
  Rate Transition31/1 -> Pack1/52(waterDepth)

== system code_gen_man_bin/Actuator Outputs/To Drive Motor ==
  identifier : Inport  OutDataType=sfix(16)  OutScaling=2^0
  data : Inport  Port=2  OutDataType=sfix(16)  OutScaling=2^0
  data_length : Inport  Port=3  OutDataType=sfix(16)  OutScaling=2^0
  trigger : Inport  Port=4
  C-function Call : Subsystem
  Constant : Constant  Value=buffer  OutDataTypeMode=uint8  OutDataType=sfix(16)  OutScaling=2^0  OutDataTypeStr=uint8
  Constant2 : Constant  Value=ide  OutDataTypeMode=uint8  OutDataType=sfix(16)  OutScaling=2^0  OutDataTypeStr=uint8
  Constant3 : Constant  Value=remote  OutDataTypeMode=uint8  OutDataType=sfix(16)  OutScaling=2^0  OutDataTypeStr=uint8
  Extract Bits : simulink/Logic and Bit Operations/Extract Bits  SystemSampleTime=-1  bitsToExtract=Upper half  numBits=8  bitIdxRange=[0 7]  outScalingMode=Treat bit field as an integer
  Extract Bits1 : simulink/Logic and Bit Operations/Extract Bits  SystemSampleTime=-1  bitsToExtract=Lower half  numBits=8  bitIdxRange=[0 7]  outScalingMode=Preserve fixed-point scaling
  myMux : Stateflow chart  TreatAsAtomicUnit=on
  uint8 combiner1 : Subsystem
  uint8 combiner2 : Subsystem
  wires:
  trigger/1 -> C-function Call/Enable
  myMux/1(y) -> C-function Call/1(parameters)
  uint8 combiner2/1(combined) -> myMux/1(u1)
  Constant/1 -> uint8 combiner2/1(high-order)
  data_length/1 -> uint8 combiner2/2(low-order)
  Extract Bits/1 -> myMux/3(u3)
  Extract Bits1/1 -> myMux/2(u2)
  identifier/1 -> Extract Bits1/1, Extract Bits/1
  uint8 combiner1/1(combined) -> myMux/4(u4)
  Constant3/1 -> uint8 combiner1/2(low-order)
  Constant2/1 -> uint8 combiner1/1(high-order)
  data/1 -> myMux/5(u5)

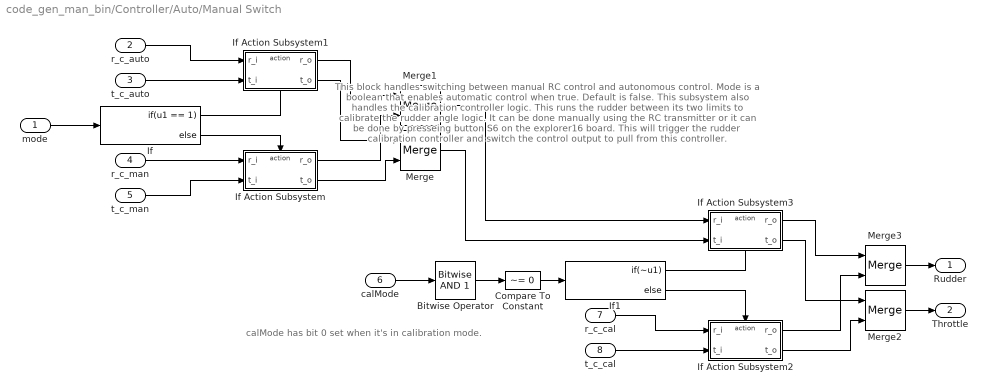
== system code_gen_man_bin/Controller/Auto/Manual Switch ==
  note: This block handles switching between manual RC control and autonomous control.
      | Mode is a boolean that enables automatic control when true. Default is false.
      |
      | This subsystem also handles the calibration controller logic. This runs the rudder between
      | its two limits to calibrate the rudder angle logic. It can be done manually using the RC
      | transmitter or it can be done by presseing button S6 on the explorer16 board. This will
      | trigger the rudder calibration controller and switch the control output to pull from this
      | controller.
  note: calMode has bit 0 set when it's in
      | calibration mode.
  mode : Inport
  r_c_auto : Inport  Port=2
  t_c_auto : Inport  Port=3
  r_c_man : Inport  Port=4
  t_c_man : Inport  Port=5
  calMode : Inport  Port=6
  r_c_cal : Inport  Port=7
  t_c_cal : Inport  Port=8
  Bitwise Operator : simulink/Logic and Bit Operations/Bitwise Operator  logicop=AND  UseBitMask=on  BitMask=1  BitMaskRealWorld=Stored Integer
  Compare To Constant : simulink/Logic and Bit Operations/Compare To Constant  SystemSampleTime=-1  relop=~=  const=0  LogicOutDataTypeMode=boolean
  If : If  IfExpression=u1 == 1
  If Action Subsystem : Subsystem  TreatAsAtomicUnit=on
  If Action Subsystem1 : Subsystem  TreatAsAtomicUnit=on
  If Action Subsystem2 : Subsystem  TreatAsAtomicUnit=on
  If Action Subsystem3 : Subsystem  TreatAsAtomicUnit=on
  If1 : If  IfExpression=~u1
  Merge{,1..3} (4 alike) : Merge
  Rudder : Outport
  Throttle : Outport  Port=2
  wires:
  If/1 -> If Action Subsystem1/Action
  If/2 -> If Action Subsystem/Action
  mode/1 -> If/1
  t_c_auto/1 -> If Action Subsystem1/2(t_i)
  r_c_auto/1 -> If Action Subsystem1/1(r_i)
  r_c_man/1 -> If Action Subsystem/1(r_i)
  t_c_man/1 -> If Action Subsystem/2(t_i)
  If Action Subsystem1/1(r_o) -> Merge1/1
  If Action Subsystem1/2(t_o) -> Merge/1
  If Action Subsystem/1(r_o) -> Merge1/2
  If Action Subsystem/2(t_o) -> Merge/2
  Merge1/1 -> If Action Subsystem3/1(r_i)
  Merge/1 -> If Action Subsystem3/2(t_i)
  If1/1 -> If Action Subsystem3/Action
  If1/2 -> If Action Subsystem2/Action
  If Action Subsystem3/1(r_o) -> Merge3/1
  If Action Subsystem3/2(t_o) -> Merge2/1
  If Action Subsystem2/1(r_o) -> Merge3/2
  If Action Subsystem2/2(t_o) -> Merge2/2
  Merge3/1 -> Rudder/1
  Merge2/1 -> Throttle/1
  r_c_cal/1 -> If Action Subsystem2/1(r_i)
  t_c_cal/1 -> If Action Subsystem2/2(t_i)
  calMode/1 -> Bitwise Operator/1
  Bitwise Operator/1 -> Compare To Constant/1
  Compare To Constant/1 -> If1/1

== system code_gen_man_bin/Controller/Autonomous Controller ==
  note: This subsystem currently provides autonomous control of the boat. It utilizes simple PID control
      | on the throttle and rudder based on desired location and bearing. Calculations are performed
      | to compute a straight-line path between current location and the programmed waypoint. The
      | boat then sets out to achieve this course.
  GPS : Inport  OutDataType=sfix(16)  OutScaling=2^0
  sensors_t : Inport  Port=2  OutDataType=sfix(16)  OutScaling=2^0
  sensors_r : Inport  Port=3  OutDataType=sfix(16)  OutScaling=2^0
  sensors_b : Inport  Port=4  OutDataType=sfix(16)  OutScaling=2^0
  reset : Inport  Port=5  OutDataType=sfix(16)  OutScaling=2^0
  waypoints : Inport  Port=6  OutDataType=sfix(16)  OutScaling=2^0
  Ballast Command : Subsystem
  Bus Selector : BusSelector  OutputSignals=sog
  Rudder Command : Subsystem
  State Keeper & Estimator : Subsystem
  Terminator : Terminator
  Terminator1 : Terminator
  Terminator2 : Terminator
  Throttle Command : Subsystem
  Rudder command : Outport  OutDataType=sfix(16)  OutScaling=2^0
  Throttle command : Outport  Port=2  OutDataType=sfix(16)  OutScaling=2^0
  Tray angle command : Outport  Port=3  OutDataType=sfix(16)  OutScaling=2^0
  tag scope: waypoints=global
  wires:
  Bus Selector/1 -> Rudder Command/5(Speed)  "<sog>"
  State Keeper & Estimator/8(datetime) -> Terminator1/1
  State Keeper & Estimator/7(lla) -> Terminator/1
  State Keeper & Estimator/3(sensors_b) -> Terminator2/1
  sensors_t/1 -> State Keeper & Estimator/1(throttle)
  sensors_r/1 -> State Keeper & Estimator/2(rudder)
  sensors_b/1 -> State Keeper & Estimator/5(ballast)
  Ballast Command/1(c_ballast) -> Tray angle command/1
  Rudder Command/1(Command) -> Rudder command/1
  Throttle Command/1(command) -> Throttle command/1
  GPS/1 -> Bus Selector/1, State Keeper & Estimator/4(gps)
  State Keeper & Estimator/4(velocity) -> Rudder Command/1(Velocity)
  State Keeper & Estimator/2(sensors_r) -> Rudder Command/2(Sensors)
  State Keeper & Estimator/1(sensors_t) -> Throttle Command/1(sensors)
  State Keeper & Estimator/5(pos) -> Rudder Command/4(Local pos)
  reset/1 -> State Keeper & Estimator/3(reset), Throttle Command/2(reset), Rudder Command/3(Reset)
  waypoints/1 -> [waypoints]

== system code_gen_man_bin/Controller/RC Inputs ==
  note: Here we only enable manual control of the vehicle if we've already calibrated.
  manual_r : Inport
  manual_t : Inport  Port=2
  rudderAngle : Inport  Port=3
  Compare To Constant : simulink/Logic and Bit Operations/Compare To Constant  SystemSampleTime=-1  relop===  const=3  LogicOutDataTypeMode=boolean
  Map PWM values to Actuator Signals : Subsystem
  command_r : Outport
  command_t : Outport  Port=2
  wires:
  manual_r/1 -> Map PWM values to Actuator Signals/1(rCmd)
  Map PWM values to Actuator Signals/1(Out1) -> command_r/1
  Map PWM values to Actuator Signals/2(Out2) -> command_t/1
  manual_t/1 -> Map PWM values to Actuator Signals/2(tCmd)
  [calibrationState] -> Compare To Constant/1
  Compare To Constant/1 -> Map PWM values to Actuator Signals/Enable
  rudderAngle/1 -> Map PWM values to Actuator Signals/3(rAngle)
